simulink model "State_UA_Khoo"  (Simulink 7.0)
settings: Solver=ode45  StartTime=0.0  StopTime=10.0  RelTol=1e-3
values from neighbouring files (symbols this model uses):
  R_CW = 1.03    [Pleural_Schuessler_IC.m]    (also in Pmus_Flow_Younes_IC.m; Resp_Mech_IC.m; Respiratory_IC.m)
  R_L = 1.69    [Pleural_Schuessler_IC.m]    (also in Pmus_Flow_Younes_IC.m; Resp_Mech_IC.m; Respiratory_IC.m)
undefined symbols (not defined in the file or in its folder): A_0_ua, Arousal_UAIC, b_ua, C_ua_awake, K_ua, R_LAW, R_trachea
settings Model: Creator=CLM  LastModifiedBy=CLM
settings OptimizationCC: BlockReduction=off  BooleanDataType=off
settings DebuggingCC: SaveWithParameterizedLinksMsg=none  SignalResolutionControl=TryResolveAllWithWarning  SolverPrmCheckMsg=none  MultiTaskDSMMsg=warning  MultiTaskCondExecSysMsg=none  StrictBusMsg=None
settings HardwareCC: TargetUnknown=on
settings RTWCC: IncludeERTFirstTime=on
settings GRTTargetCC: TargetFcnLib=ansi_tfl_tmw.mat

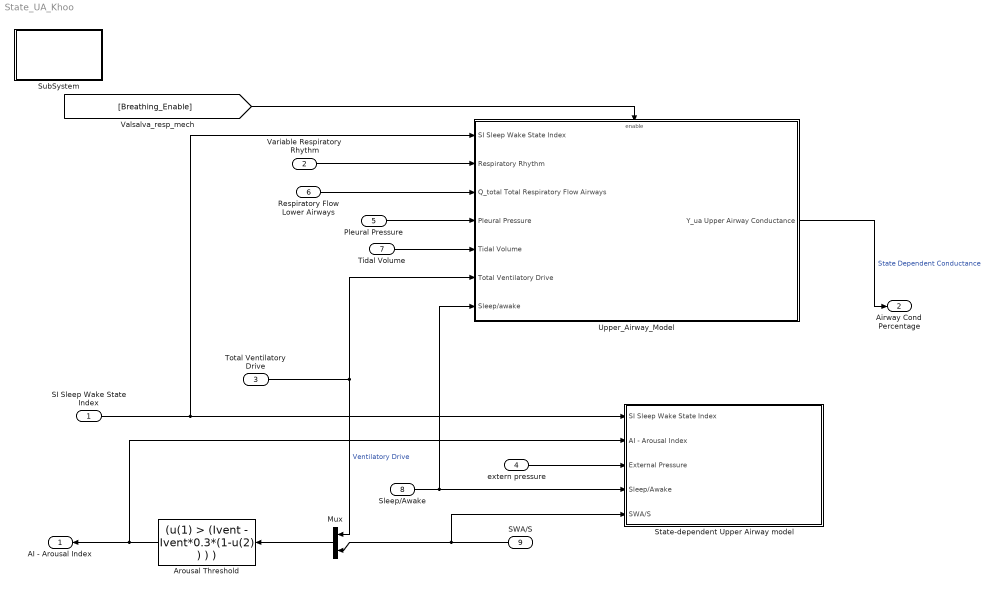
== system State_UA_Khoo ==
  SI Sleep Wake State Index : Inport  OutDataType=sfix(16)  OutScaling=2^0
  Variable Respiratory Rhythm : Inport  Port=2  OutDataType=sfix(16)  OutScaling=2^0
  Total Ventilatory Drive : Inport  Port=3  OutDataType=sfix(16)  OutScaling=2^0
  extern pressure : Inport  Port=4  OutDataType=sfix(16)  OutScaling=2^0
  Pleural Pressure : Inport  Port=5  OutDataType=sfix(16)  OutScaling=2^0
  Respiratory Flow Lower Airways : Inport  Port=6  OutDataType=sfix(16)  OutScaling=2^0
  Tidal Volume : Inport  Port=7  OutDataType=sfix(16)  OutScaling=2^0
  Sleep/Awake : Inport  Port=8  OutDataType=sfix(16)  OutScaling=2^0
  SWA/S : Inport  Orientation=left  Port=9  OutDataType=sfix(16)  OutScaling=2^0
  Arousal Threshold : Fcn  Orientation=left  Expr=(u(1) > (Ivent - Ivent*0.3*(1-u(2) ) ) )
  Mux : Mux  Orientation=left  Inputs=2
  State-dependent Upper Airway model : Subsystem
  SubSystem : Subsystem
      settings: OpenFcn=State_UA_Khoo_IC
      mask Display: disp('"double click here"\n to load \nState_UA_Khoo \ninitial values');
  Upper_Airway_Model : Subsystem  TreatAsAtomicUnit=on
  AI - Arousal Index : Outport  Orientation=left  OutDataType=sfix(16)  OutScaling=2^0
  "Airway Cond Percentage " : Outport  Port=2  OutDataType=sfix(16)  OutScaling=2^0
  wires:
  SI Sleep Wake State Index/1 -> Upper_Airway_Model/1(SI Sleep Wake State Index), State-dependent Upper Airway model/1(SI Sleep Wake State Index)
  extern pressure/1 -> State-dependent Upper Airway model/3(External Pressure)
  SWA/S/1 -> Mux/2, State-dependent Upper Airway model/5(SWA/S)
  Total Ventilatory Drive/1 -> Upper_Airway_Model/6(Total Ventilatory Drive), Mux/1  "Ventilatory Drive"
  Sleep/Awake/1 -> State-dependent Upper Airway model/4(Sleep/Awake), Upper_Airway_Model/7(Sleep/awake)
  Upper_Airway_Model/1("Y_ua Upper Airway Conductance ") -> "Airway Cond Percentage "/1  "State Dependent Conductance"
  Variable Respiratory Rhythm/1 -> Upper_Airway_Model/2(Respiratory Rhythm)
  Respiratory Flow Lower Airways/1 -> Upper_Airway_Model/3(Q_total Total Respiratory Flow Airways)
  Pleural Pressure/1 -> Upper_Airway_Model/4(Pleural Pressure)
  Tidal Volume/1 -> Upper_Airway_Model/5(Tidal Volume)
  [Breathing_Enable] -> Upper_Airway_Model/Enable
  Mux/1 -> Arousal Threshold/1
  Arousal Threshold/1 -> AI - Arousal Index/1, State-dependent Upper Airway model/2(AI - Arousal Index)

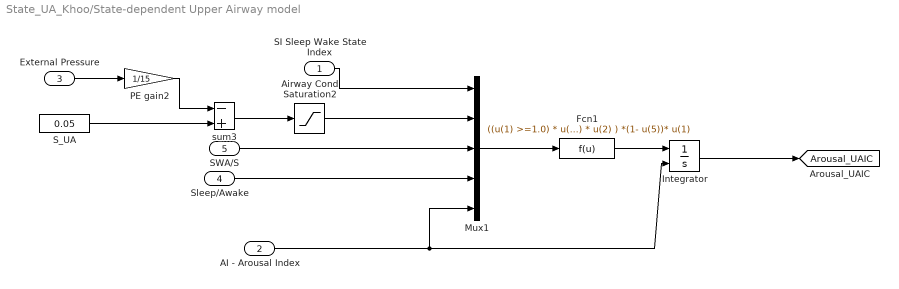
== system State_UA_Khoo/State-dependent Upper Airway model ==
  SI Sleep Wake State Index : Inport  OutDataType=sfix(16)  OutScaling=2^0
  AI - Arousal Index : Inport  Port=2  OutDataType=sfix(16)  OutScaling=2^0
  External Pressure : Inport  Port=3  OutDataType=sfix(16)  OutScaling=2^0
  Sleep/Awake : Inport  Port=4  OutDataType=sfix(16)  OutScaling=2^0
  SWA/S : Inport  Port=5  OutDataType=sfix(16)  OutScaling=2^0
  Airway Cond Saturation2 : Saturate  UpperLimit=1  LowerLimit=0
  Fcn1 : Fcn  Expr="((u(1) >=1.0) * u(2) * (1 + 0.3 * (1 - u(3)) * (1-u(4)) )  + ( u(1)<1.0) * u(1) * u(2) ) *(1- u(5))* u(1)"
  Integrator : Integrator  ExternalReset=rising  InitialCondition=Arousal_UAIC
  Mux1 : Mux  Inputs=5
  PE gain2 : Gain  Gain=1/15  ParameterDataType=sfix(16)  ParameterScaling=2^0  OutDataType=sfix(16)  OutScaling=2^0  SaturateOnIntegerOverflow=on
  S_UA : Constant  Value=0.05  OutDataType=sfix(16)  OutScaling=2^0
  sum3 : Sum  Inputs=-+  OutDataType=sfix(16)  OutScaling=2^0  SaturateOnIntegerOverflow=on  InputSameDT=on
  tag scope: Arousal_UAIC=global
  wires:
  AI - Arousal Index/1 -> Integrator/2, Mux1/5
  SI Sleep Wake State Index/1 -> Mux1/1
  SWA/S/1 -> Mux1/3
  Sleep/Awake/1 -> Mux1/4
  S_UA/1 -> sum3/2
  sum3/1 -> Airway Cond Saturation2/1
  External Pressure/1 -> PE gain2/1
  PE gain2/1 -> sum3/1
  Mux1/1 -> Fcn1/1
  Airway Cond Saturation2/1 -> Mux1/2
  Fcn1/1 -> Integrator/1
  Integrator/1 -> [Arousal_UAIC]

== system State_UA_Khoo/SubSystem ==

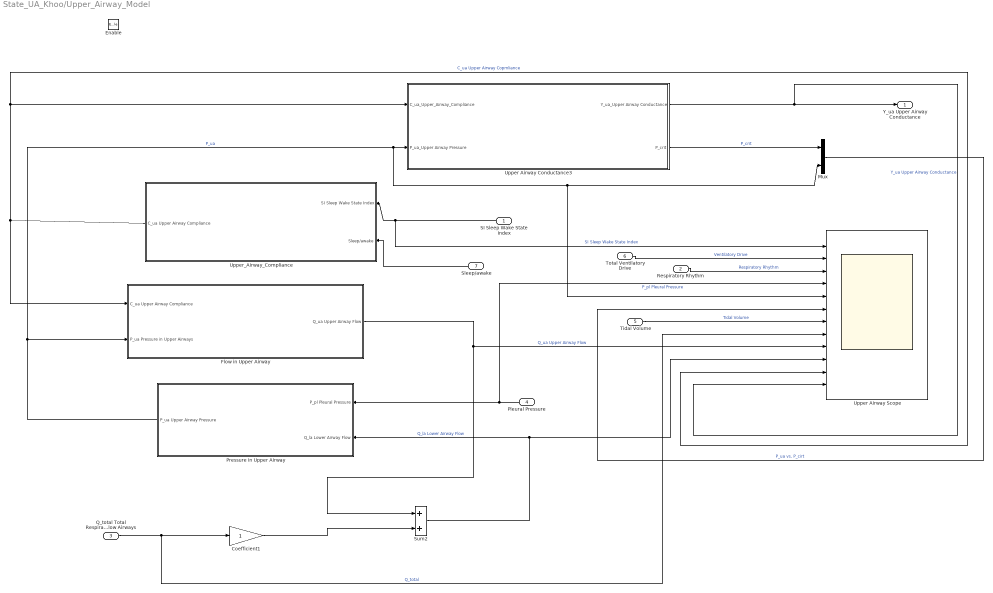
== system State_UA_Khoo/Upper_Airway_Model ==
  SI Sleep Wake State Index : Inport  Orientation=left  OutDataType=sfix(16)  OutScaling=2^0
  Respiratory Rhythm : Inport  Port=2  OutDataType=sfix(16)  OutScaling=2^0
  Q_total Total Respiratory Flow Airways : Inport  Port=3  OutDataType=sfix(16)  OutScaling=2^0
  Pleural Pressure : Inport  Orientation=left  Port=4  OutDataType=sfix(16)  OutScaling=2^0
  Tidal Volume : Inport  Port=5  OutDataType=sfix(16)  OutScaling=2^0
  Total Ventilatory Drive : Inport  Port=6  OutDataType=sfix(16)  OutScaling=2^0
  Sleep/awake : Inport  Orientation=left  Port=7  OutDataType=sfix(16)  OutScaling=2^0
  Enable : EnablePort
  " Flow in Upper Airway" : Subsystem
  " Pressure in Upper Airway" : Subsystem  Orientation=left
  Coefficient1 : Gain  ParameterDataType=sfix(16)  ParameterScaling=2^0  OutDataType=sfix(16)  OutScaling=2^0  SaturateOnIntegerOverflow=on
  Mux : Mux  Inputs=2
  Sum2 : Sum  OutDataType=sfix(16)  OutScaling=2^0  SaturateOnIntegerOverflow=on
  Upper Airway Conductance3 : Subsystem
  Upper Airway Scope : Scope  NumInputPorts=12
      settings: TimeRange=120  YMin=0~0.2~-0.05~-40~-4~-41~-0.1~-2~-2e-006~-4~0.005~0.5  YMax=1~0.48~1.05~5~1.5~10~3~2.5~5e-006~5~0.01~1.05  SaveName=ScopeData20  MaxDataPoints=50
  Upper_Airway_Compliance : Subsystem  Orientation=left
  "Y_ua Upper Airway Conductance " : Outport  OutDataType=sfix(16)  OutScaling=2^0  InitialOutput=[0]
  wires:
  Q_total Total Respiratory Flow Airways/1 -> Upper Airway Scope/8, Coefficient1/1  "Q_total"
  SI Sleep Wake State Index/1 -> Upper_Airway_Compliance/1("SI Sleep Wake State Index "), Upper Airway Scope/1  "SI Sleep Wake State Index"
  Pleural Pressure/1 -> Upper Airway Scope/4, " Pressure in Upper Airway"/1(P_pl Pleural Pressure)  "P_pl Pleural Pressure"
  Sum2/1 -> " Pressure in Upper Airway"/2(Q_la Lower Airway Flow), Upper Airway Scope/10  "Q_la Lower Airway Flow"
  " Pressure in Upper Airway"/1("P_ua Upper Airway Pressure ") -> " Flow in Upper Airway"/2(P_ua Pressure in Upper Airways), Upper Airway Conductance3/2(P_ua_Upper Airway Pressure), Mux/2, Upper Airway Scope/5  "P_ua"
  Upper Airway Conductance3/2(P_crit) -> Mux/1  "P_crit"
  Upper_Airway_Compliance/1(C_ua Upper Airway Compliance) -> " Flow in Upper Airway"/1(C_ua Upper Airway Compliance), Upper Airway Conductance3/1(C_ua_Upper_Airway_Compliance), Upper Airway Scope/11  "C_ua Upper Airway Copmliance"
  " Flow in Upper Airway"/1("Q_ua Upper Airway Flow ") -> Upper Airway Scope/9, Sum2/1  "Q_ua Upper Airway Flow"
  Upper Airway Conductance3/1(Y_ua_Upper Airway Conductance) -> Upper Airway Scope/12, "Y_ua Upper Airway Conductance "/1  "Y_ua Upper Airway Conductance"
  Total Ventilatory Drive/1 -> Upper Airway Scope/2  "Ventilatory Drive"
  Mux/1 -> Upper Airway Scope/6  "P_ua vs. P_cirt"
  Tidal Volume/1 -> Upper Airway Scope/7  "Tidal Volume"
  Respiratory Rhythm/1 -> Upper Airway Scope/3  "Respiratory Rhythm"
  Sleep/awake/1 -> Upper_Airway_Compliance/2(Sleep/awake)
  Coefficient1/1 -> Sum2/2

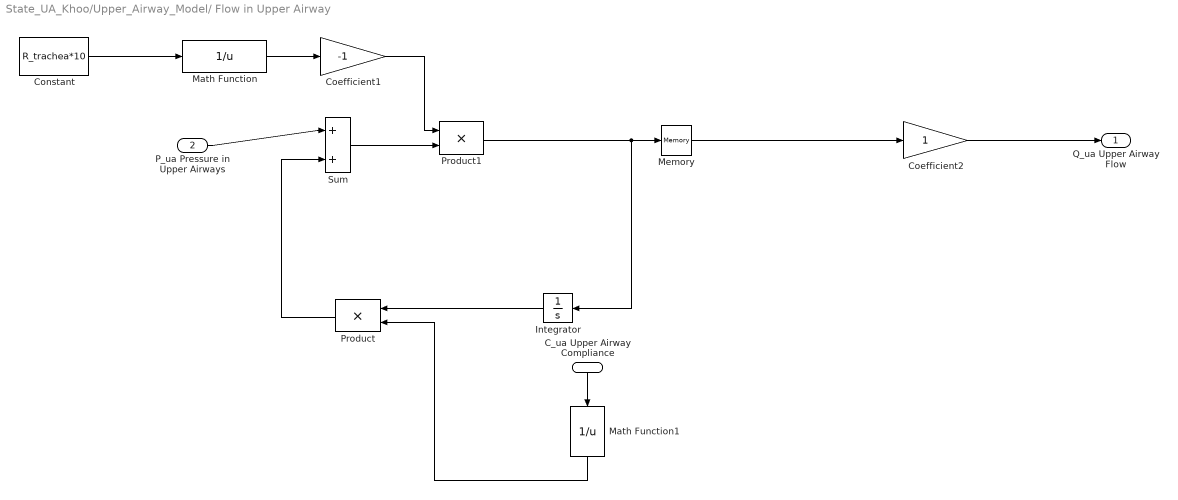
== system State_UA_Khoo/Upper_Airway_Model/ Flow in Upper Airway ==
  C_ua Upper Airway Compliance : Inport  Orientation=down  OutDataType=sfix(16)  OutScaling=2^0
  P_ua Pressure in Upper Airways : Inport  Port=2  OutDataType=sfix(16)  OutScaling=2^0
  Coefficient1 : Gain  Gain=-1  ParameterDataType=sfix(16)  ParameterScaling=2^0  OutDataType=sfix(16)  OutScaling=2^0  SaturateOnIntegerOverflow=on
  Coefficient2 : Gain  ParameterDataType=sfix(16)  ParameterScaling=2^0  OutDataType=sfix(16)  OutScaling=2^0  SaturateOnIntegerOverflow=on
  Constant : Constant  Value=R_trachea*10  OutDataType=sfix(16)  OutScaling=2^0
  Integrator : Integrator  Orientation=left  LimitOutput=on  UpperSaturationLimit=100  LowerSaturationLimit=-100
  Math Function : Math  Operator=reciprocal  OutDataType=sfix(16)  OutScaling=2^0  SaturateOnIntegerOverflow=on
  Math Function1 : Math  Orientation=down  Operator=reciprocal  OutDataType=sfix(16)  OutScaling=2^0  SaturateOnIntegerOverflow=on
  Memory : Memory
  Product : Product  Orientation=left  OutDataType=sfix(16)  OutScaling=2^0  SaturateOnIntegerOverflow=on
  Product1 : Product  OutDataType=sfix(16)  OutScaling=2^0  SaturateOnIntegerOverflow=on
  Sum : Sum  Inputs=|++  OutDataType=sfix(16)  OutScaling=2^0  SaturateOnIntegerOverflow=on
  "Q_ua Upper Airway Flow " : Outport  OutDataType=sfix(16)  OutScaling=2^0
  wires:
  Product1/1 -> Integrator/1, Memory/1
  P_ua Pressure in Upper Airways/1 -> Sum/1
  Sum/1 -> Product1/2
  C_ua Upper Airway Compliance/1 -> Math Function1/1
  Integrator/1 -> Product/1
  Product/1 -> Sum/2
  Constant/1 -> Math Function/1
  Math Function/1 -> Coefficient1/1
  Coefficient1/1 -> Product1/1
  Coefficient2/1 -> "Q_ua Upper Airway Flow "/1
  Memory/1 -> Coefficient2/1
  Math Function1/1 -> Product/2

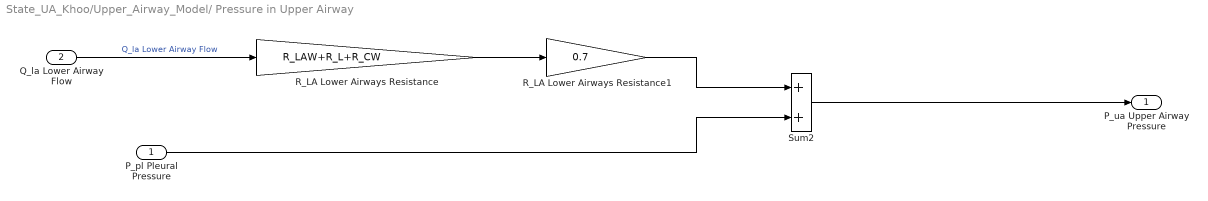
== system State_UA_Khoo/Upper_Airway_Model/ Pressure in Upper Airway ==
  P_pl Pleural Pressure : Inport  OutDataType=sfix(16)  OutScaling=2^0
  Q_la Lower Airway Flow : Inport  Port=2  OutDataType=sfix(16)  OutScaling=2^0
  R_LA Lower Airways Resistance : Gain  Gain=R_LAW+R_L+R_CW  ParameterDataType=sfix(16)  ParameterScaling=2^0  OutDataType=sfix(16)  OutScaling=2^0  SaturateOnIntegerOverflow=on
  R_LA Lower Airways Resistance1 : Gain  Gain=0.7  ParameterDataType=sfix(16)  ParameterScaling=2^0  OutDataType=sfix(16)  OutScaling=2^0  SaturateOnIntegerOverflow=on
  Sum2 : Sum  OutDataType=sfix(16)  OutScaling=2^0  SaturateOnIntegerOverflow=on
  "P_ua Upper Airway Pressure " : Outport  OutDataType=sfix(16)  OutScaling=2^0  InitialOutput=[0]
  wires:
  Q_la Lower Airway Flow/1 -> R_LA Lower Airways Resistance/1  "Q_la Lower Airway Flow"
  P_pl Pleural Pressure/1 -> Sum2/2
  Sum2/1 -> "P_ua Upper Airway Pressure "/1
  R_LA Lower Airways Resistance/1 -> R_LA Lower Airways Resistance1/1
  R_LA Lower Airways Resistance1/1 -> Sum2/1

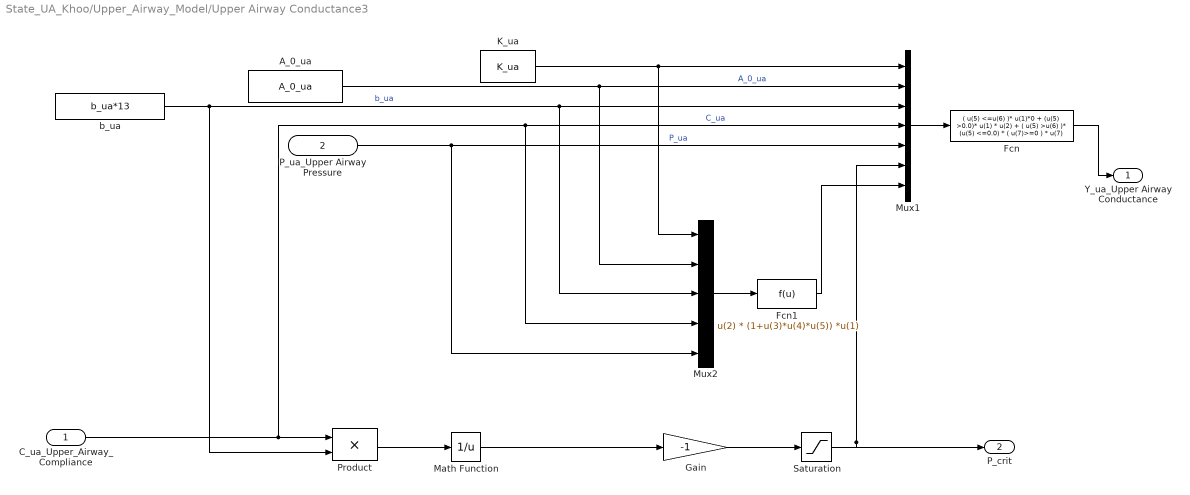
== system State_UA_Khoo/Upper_Airway_Model/Upper Airway Conductance3 ==
  C_ua_Upper_Airway_Compliance : Inport  OutDataType=sfix(16)  OutScaling=2^0
  P_ua_Upper Airway Pressure : Inport  Port=2  OutDataType=sfix(16)  OutScaling=2^0
  A_0_ua : Constant  Value=A_0_ua  OutDataType=sfix(16)  OutScaling=2^0
  Fcn : Fcn  Expr="( u(5) <=u(6) )* u(1)*0  + (u(5) >0.0)* u(1) * u(2) +  ( u(5) >u(6) )* (u(5) <=0.0) * ( u(7)>=0 ) * u(7)"
  Fcn1 : Fcn  Expr=u(2) * (1+u(3)*u(4)*u(5)) *u(1)
  Gain : Gain  Gain=-1  ParameterDataType=sfix(16)  ParameterScaling=2^0  OutDataType=sfix(16)  OutScaling=2^0  SaturateOnIntegerOverflow=on
  K_ua : Constant  Value=K_ua  OutDataType=sfix(16)  OutScaling=2^0
  Math Function : Math  Operator=reciprocal  OutDataType=sfix(16)  OutScaling=2^0  SaturateOnIntegerOverflow=on
  Mux1 : Mux  Inputs=7
  Mux2 : Mux  Inputs=5
  Product : Product  OutDataType=sfix(16)  OutScaling=2^0  SaturateOnIntegerOverflow=on
  Saturation : Saturate  UpperLimit=10  LowerLimit=-40
  b_ua : Constant  Value=b_ua*13  OutDataType=sfix(16)  OutScaling=2^0
  Y_ua_Upper Airway Conductance : Outport  OutDataType=sfix(16)  OutScaling=2^0
  P_crit : Outport  Port=2  OutDataType=sfix(16)  OutScaling=2^0
  wires:
  P_ua_Upper Airway Pressure/1 -> Mux1/5, Mux2/5  "P_ua"
  K_ua/1 -> Mux1/1, Mux2/1
  C_ua_Upper_Airway_Compliance/1 -> Mux1/4, Mux2/4, Product/1  "C_ua"
  b_ua/1 -> Mux1/3, Mux2/3, Product/2  "b_ua"
  A_0_ua/1 -> Mux1/2, Mux2/2  "A_0_ua"
  Mux1/1 -> Fcn/1
  Fcn/1 -> Y_ua_Upper Airway Conductance/1
  Fcn1/1 -> Mux1/7
  Mux2/1 -> Fcn1/1
  Gain/1 -> Saturation/1
  Product/1 -> Math Function/1
  Math Function/1 -> Gain/1
  Saturation/1 -> P_crit/1, Mux1/6

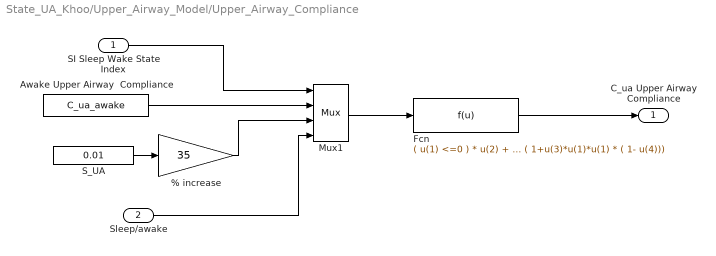
== system State_UA_Khoo/Upper_Airway_Model/Upper_Airway_Compliance ==
  "SI Sleep Wake State Index " : Inport  OutDataType=sfix(16)  OutScaling=2^0
  Sleep/awake : Inport  Port=2  OutDataType=sfix(16)  OutScaling=2^0
  % increase : Gain  Gain=35  ParameterDataType=sfix(16)  ParameterScaling=2^0  OutDataType=sfix(16)  OutScaling=2^0  SaturateOnIntegerOverflow=on
  Awake Upper Airway  Compliance : Constant  Value=C_ua_awake  OutDataType=sfix(16)  OutScaling=2^0
  Fcn : Fcn  Expr="( u(1) <=0 ) * u(2) + ( u(1) >=1) * u(2) * ( 1+u(3) ) +  ( u(1) >0 ) * ( u(1) <1 ) * u(2) * ( 1+u(3)*u(1)*u(1) * ( 1- u(4)))"
  Mux1 : Mux
  S_UA : Constant  Value=0.01  OutDataType=sfix(16)  OutScaling=2^0
  C_ua Upper Airway Compliance : Outport  OutDataType=sfix(16)  OutScaling=2^0
  wires:
  Awake Upper Airway  Compliance/1 -> Mux1/2
  "SI Sleep Wake State Index "/1 -> Mux1/1
  % increase/1 -> Mux1/3
  Mux1/1 -> Fcn/1
  Fcn/1 -> C_ua Upper Airway Compliance/1
  S_UA/1 -> % increase/1
  Sleep/awake/1 -> Mux1/4
